simulink model "sampleModel1913_sub"  (R2023a)
settings: Solver=VariableStepAuto  StartTime=0.0  StopTime=10.0  RelTol=1e-3
libraries: hdlsllib x4, simulink x4
settings Model: Creator=user1  LastModifiedBy=user1
settings OptimizationCC: BlockReduction=off  ConditionallyExecuteInputs=off

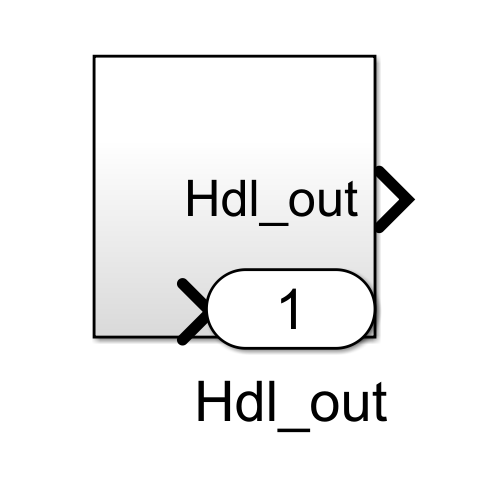
[thumbnail: Simulink's stored preview of the top-level diagram]
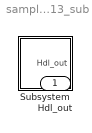
== system sampleModel1913_sub ==
  Subsystem : Subsystem
  Hdl_out : Outport  OutDataTypeStr=uint8

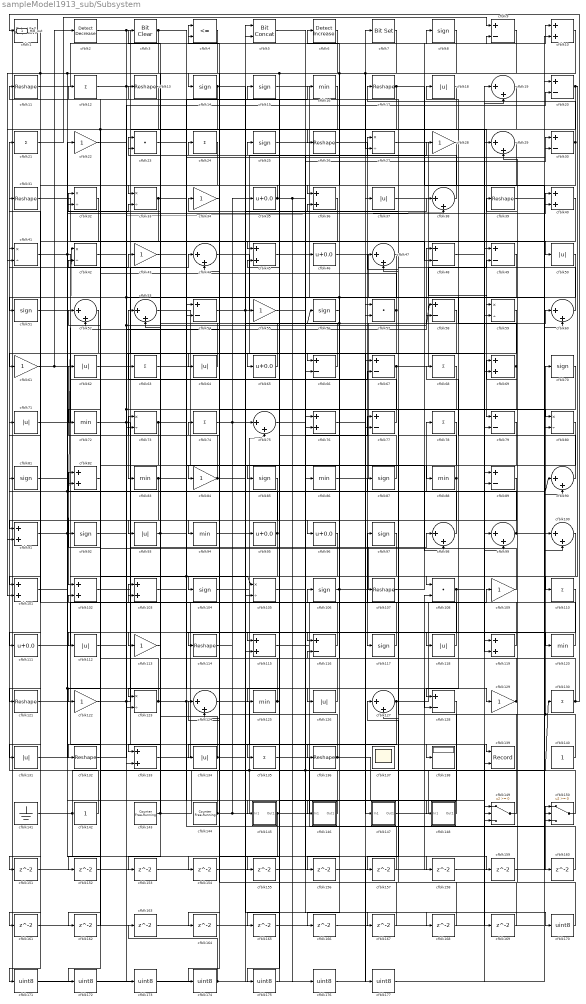
== system sampleModel1913_sub/Subsystem ==
  cfblk1 : hdlsllib/Logic and Bit Operations/Detect Fall Nonpositive  vinit=0  OutDataTypeStr=uint8
  cfblk{10,36,40,45,69,76,82,91,101..103,115,119,133} (14 alike) : Sum  OutDataTypeStr=uint8
  cfblk{19,29,38,44,47,52..53,60,75,90,98..100,124,127} (15 alike) : Sum  Inputs=|++  OutDataTypeStr=uint8
  cfblk{8,14..15,25,51,56,70,81,85,87,92,97,104,106,117} (15 alike) : Signum
  cfblk{27,32..33,41..42,59,73,80,105,123} (10 alike) : Product  Inputs=*/  OutDataTypeStr=uint8  RndMeth=Zero  SaturateOnIntegerOverflow=on
  cfblk{11,13,17,26,31,39,107,114,121,132,136} (11 alike) : Reshape
  cfblk108 : DotProduct  OutDataTypeStr=uint8
  cfblk{22,28,34,43,55,61,84,109,113,122,129} (11 alike) : Gain  OutDataTypeStr=uint8
  cfblk{12,21,24,63,68,74,78,110,130,135} (10 alike) : Sum  Inputs=+  OutDataTypeStr=uint8
  cfblk{35,46,65,95..96,111} (6 alike) : Bias  Bias=0.0  SaturateOnIntegerOverflow=off
  cfblk{18,37,50,62,64,71,93,112,118,126,131,134} (12 alike) : Abs  OutDataTypeStr=uint8  SaturateOnIntegerOverflow=off
  cfblk{9,20,30,48..49,54,58,66..67,77,79,89,116,128} (14 alike) : Sum  Inputs=+-  OutDataTypeStr=uint8
  cfblk{16,72,83,86,88,94,120,125} (8 alike) : MinMax  OutDataTypeStr=uint8
  cfblk137 : Scope
      settings: Floating=on
  cfblk138 : Display
  cfblk139 : Record  FileSettingsInternal="{\"entries\":[{\"content\":{\"excelSettings\":{\"content\":{},\"type\":\"Streamout.ExcelSettings\"}},\"type\":\"Streamout.FileSettingStorage\",\"uuid\":\"\"}],\"packageUris\":[\"http:\\/\\/schema.mathworks.com\\/mf0\\/streamout_blocks\\/R2020a\"],\"version\":\"1.0\"}"  Layout=[1 1]  SignalsInternal="{\"entries\":[{\"content\":{\"signals\":[{\"content\":{\"blockPath\":[],\"dimensions\":[1],\"domain\":\"\",\"lineColor\":\"#a2142f\",\"plots\":[1],\"port\":1,\"signalID\":51559,\"signalName\":\"cfblk72\"},\"type\":\"RecordBlkView.Signal\",\"uuid\":\"\"},{\"content\":{\"blockPath\":[],\"dimensions\":[1],\"domain\":\"\",\"lineColor\":\"#139fff\",\"plots\":[1],\"port\":2,\"signalID\":51562,\"signalName\":\"cfblk92\"},\"type\":\"RecordBlkView.Signal\",\"uuid\":\"\"}]},\"type\":\"RecordBlkView.InputSignals\",\"uuid\":\"\"}],\"packageUris\":[\"http:\\/\\/schema.mathworks.com\\/mf0\\/streamout_blocks\\/R2020a\"],\"version\":\"1.0\"}"  VisualizationBindings="{\"xyplotplugin\":{\"info\":[{\"series\":[{\"bindingParametersList\":[{\"parameter\":\"X-Axis\",\"signalID\":51559,\"signalName\":\"cfblk72\"},{\"parameter\":\"Y-Axis\",\"signalID\":51562,\"signalName\":\"cfblk92\"}],\"seriesID\":58635}],\"subplotID\":1}]}}"  CompatibilityTag=XY  st=-1
  cfblk140 : Constant  OutDataTypeStr=uint8  SampleTime=-1
  cfblk141 : Ground
  cfblk142 : Constant  OutDataTypeStr=uint8  SampleTime=-1
  cfblk143 : hdlsllib/Sources/Counter Free-Running  NumBits=16  tsamp=-1
  cfblk144 : hdlsllib/Sources/Counter Free-Running  NumBits=16  tsamp=-1
  cfblk145 : Subsystem
      settings: LibrarySourceBlock=|
      | hdlsllib/Ports &
      | Subsystems/Subsystem
  cfblk146 : Subsystem
      settings: LibrarySourceBlock=|
      | hdlsllib/Ports &
      | Subsystems/Subsystem
  cfblk147 : Subsystem
      settings: LibrarySourceBlock=|
      | hdlsllib/Ports &
      | Subsystems/Subsystem
  cfblk148 : Subsystem
      settings: LibrarySourceBlock=|
      | hdlsllib/Ports &
      | Subsystems/Subsystem
  cfblk149 : Switch  OutDataTypeStr=uint8  SaturateOnIntegerOverflow=off  InputSameDT=off
  cfblk150 : Switch  OutDataTypeStr=uint8  SaturateOnIntegerOverflow=off  InputSameDT=off
  cfblk{151..169} (19 alike) : Delay  SampleTime=1
  cfblk{170..177} (8 alike) : DataTypeConversion  OutDataTypeStr=uint8  SaturateOnIntegerOverflow=off  RndMeth=Floor
  cfblk2 : simulink/Logic and Bit Operations/Detect Decrease  vinit=0.0  OutDataTypeStr=uint8
      settings: LibrarySourceBlock=|
      | hdlsllib/Logic and Bit
      | Operations/Detect
      | Decrease
  cfblk23 : DotProduct  OutDataTypeStr=uint8
  cfblk3 : simulink/Logic and Bit Operations/Bit Clear  iBit=0
      settings: LibrarySourceBlock=|
      | hdlsllib/Logic and Bit
      | Operations/Bit Clear
  cfblk4 : RelationalOperator  Operator=<=  OutDataTypeStr=boolean  InputSameDT=off
  cfblk5 : hdlsllib/Logic and Bit Operations/Bit Concat  numInputs=2
  cfblk57 : DotProduct  OutDataTypeStr=uint8
  cfblk6 : simulink/Logic and Bit Operations/Detect Increase  vinit=0.0  OutDataTypeStr=uint8
      settings: LibrarySourceBlock=|
      | hdlsllib/Logic and Bit
      | Operations/Detect
      | Increase
  cfblk7 : simulink/Logic and Bit Operations/Bit Set  iBit=0
      settings: LibrarySourceBlock=|
      | hdlsllib/Logic and Bit
      | Operations/Bit Set
  Hdl_out : Outport  OutDataTypeStr=uint8
  wires:
  cfblk4/1 -> cfblk14/1
  cfblk72/1 -> cfblk139/1, cfblk77/2, cfblk58/2
  cfblk2/1 -> cfblk66/1, cfblk69/2, cfblk60/2
  cfblk45/1 -> cfblk86/1
  cfblk15/1 -> cfblk108/1
  cfblk114/1 -> cfblk55/1, cfblk75/1
  cfblk142/1 -> cfblk21/1
  cfblk99/1 -> cfblk90/2, cfblk6/1, cfblk56/1
  cfblk111/1 -> cfblk106/1
  cfblk64/1 -> cfblk41/1
  cfblk30/1 -> cfblk64/1, cfblk17/1
  cfblk91/1 -> cfblk159/1, cfblk42/1
  cfblk61/1 -> cfblk2/1, cfblk104/1
  cfblk26/1 -> cfblk117/1
  cfblk41/1 -> cfblk146/1(In1), cfblk138/1
  cfblk144/1 -> cfblk92/1, cfblk35/1, cfblk130/1, cfblk75/2
  cfblk149/1 -> cfblk81/1
  cfblk32/1 -> cfblk91/1
  cfblk116/1 -> cfblk71/1
  cfblk148/1(Out1) -> cfblk34/1
  cfblk122/1 -> cfblk38/2, cfblk44/1
  cfblk121/1 -> cfblk128/2, cfblk22/1
  cfblk81/1 -> cfblk102/1
  cfblk27/1 -> cfblk79/1
  cfblk86/1 -> cfblk48/1
  cfblk38/1 -> cfblk23/1
  cfblk69/1 -> cfblk165/1, cfblk18/1
  cfblk21/1 -> cfblk9/1
  cfblk85/1 -> cfblk93/1
  cfblk101/1 -> cfblk40/1
  cfblk84/1 -> cfblk60/1, cfblk62/1
  cfblk140/1 -> cfblk116/2, cfblk70/1
  cfblk34/1 -> cfblk4/1
  cfblk43/1 -> cfblk85/1
  cfblk17/1 -> cfblk73/2, cfblk40/2
  cfblk62/1 -> cfblk65/1
  cfblk97/1 -> cfblk112/1
  cfblk12/1 -> cfblk45/1, cfblk59/1
  cfblk123/1 -> cfblk42/2, cfblk145/1(In1), cfblk126/1
  cfblk105/1 -> cfblk77/1
  cfblk65/1 -> cfblk24/1
  cfblk92/1 -> cfblk139/2
  cfblk135/1 -> cfblk150/1
  cfblk133/1 -> cfblk109/1
  cfblk25/1 -> cfblk150/2
  cfblk11/1 -> cfblk8/1
  cfblk115/1 -> cfblk120/1
  cfblk6/1 -> cfblk113/1
  cfblk95/1 -> cfblk74/1, cfblk122/1
  cfblk13/1 -> cfblk41/2, cfblk132/1
  cfblk35/1 -> cfblk33/1, cfblk176/1, cfblk30/2
  cfblk57/1 -> cfblk32/2, cfblk83/1
  cfblk113/1 -> cfblk3/1
  cfblk46/1 -> cfblk100/1
  cfblk18/1 -> cfblk123/1
  cfblk141/1 -> cfblk177/1, cfblk66/2, cfblk59/2
  cfblk100/1 -> cfblk133/1
  cfblk71/1 -> cfblk37/1
  cfblk102/1 -> cfblk57/2
  cfblk14/1 -> cfblk168/1, cfblk63/1
  cfblk145/1(Out1) -> cfblk164/1, cfblk97/1
  cfblk147/1(Out1) -> cfblk19/1
  cfblk107/1 -> cfblk9/2
  cfblk67/1 -> cfblk94/1, cfblk49/2
  cfblk96/1 -> cfblk114/1
  cfblk75/1 -> cfblk28/1
  cfblk98/1 -> cfblk78/1
  cfblk10/1 -> cfblk27/2, cfblk26/1, cfblk76/2
  cfblk103/1 -> cfblk16/1
  cfblk127/1 -> cfblk134/1, cfblk19/2
  cfblk131/1 -> cfblk90/1, cfblk43/1
  cfblk77/1 -> cfblk53/1
  cfblk31/1 -> cfblk48/2
  cfblk118/1 -> cfblk23/2
  cfblk93/1 -> cfblk153/1, cfblk67/2
  cfblk82/1 -> cfblk52/1
  cfblk83/1 -> cfblk105/2, cfblk131/1
  cfblk20/1 -> cfblk124/2, cfblk110/1
  cfblk1/1 -> cfblk61/1
  cfblk150/1 -> cfblk15/1
  cfblk28/1 -> cfblk84/1
  cfblk60/1 -> cfblk11/1
  cfblk136/1 -> cfblk169/1, cfblk52/2
  cfblk120/1 -> cfblk31/1
  cfblk108/1 -> cfblk127/2, cfblk29/1
  cfblk80/1 -> cfblk135/1
  cfblk109/1 -> cfblk12/1
  cfblk23/1 -> cfblk115/1
  cfblk36/1 -> cfblk133/2
  cfblk50/1 -> cfblk121/1
  cfblk9/1 -> cfblk36/1
  cfblk63/1 -> cfblk95/1
  cfblk3/1 -> cfblk129/1, cfblk82/2, cfblk91/2
  cfblk90/1 -> cfblk68/1
  cfblk146/1(Out1) -> cfblk82/1
  cfblk19/1 -> cfblk119/2
  cfblk70/1 -> cfblk128/1
  cfblk48/1 -> cfblk50/1
  cfblk66/1 -> cfblk32/1
  cfblk51/1 -> cfblk33/2
  cfblk106/1 -> cfblk166/1, cfblk98/1
  cfblk16/1 -> cfblk72/1
  cfblk37/1 -> cfblk99/1
  cfblk134/1 -> cfblk103/1, cfblk148/1(In1)
  cfblk129/1 -> cfblk69/1, cfblk36/2
  cfblk74/1 -> cfblk136/1
  cfblk44/1 -> cfblk147/1(In1)
  cfblk124/1 -> cfblk149/2
  cfblk88/1 -> cfblk47/2, cfblk115/2
  cfblk49/1 -> cfblk88/1
  cfblk125/1 -> cfblk45/2, cfblk73/1
  cfblk87/1 -> cfblk13/1
  cfblk132/1 -> cfblk20/2, cfblk58/1
  cfblk7/1 -> cfblk174/1
  cfblk33/1 -> cfblk30/1, cfblk123/2
  cfblk143/1 -> cfblk103/2, cfblk46/1
  cfblk53/1 -> cfblk98/2
  cfblk73/1 -> cfblk172/1, cfblk118/1, cfblk105/1
  cfblk52/1 -> cfblk101/1
  cfblk29/1 -> cfblk44/2
  cfblk94/1 -> cfblk38/1
  cfblk117/1 -> cfblk107/1
  cfblk104/1 -> cfblk10/1
  cfblk79/1 -> cfblk116/1
  cfblk130/1 -> cfblk47/1, cfblk1/1
  cfblk76/1 -> cfblk80/1
  cfblk24/1 -> cfblk51/1
  cfblk47/1 -> cfblk96/1, cfblk54/2
  cfblk126/1 -> cfblk53/2
  cfblk119/1 -> cfblk87/1
  cfblk54/1 -> cfblk79/2, cfblk27/1
  cfblk8/1 -> cfblk125/1, cfblk101/2, cfblk111/1
  cfblk58/1 -> cfblk151/1
  cfblk151/1 -> cfblk76/1
  cfblk110/1 -> cfblk152/1
  cfblk152/1 -> cfblk150/3
  cfblk153/1 -> cfblk108/2
  cfblk22/1 -> cfblk154/1
  cfblk154/1 -> cfblk119/1
  cfblk128/1 -> cfblk155/1
  cfblk155/1 -> cfblk67/1
  cfblk56/1 -> cfblk156/1
  cfblk156/1 -> cfblk49/1
  cfblk68/1 -> cfblk157/1
  cfblk157/1 -> cfblk57/1
  cfblk42/1 -> cfblk158/1
  cfblk158/1 -> cfblk149/1
  cfblk159/1 -> cfblk29/2
  cfblk39/1 -> cfblk160/1
  cfblk160/1 -> cfblk54/1
  cfblk59/1 -> cfblk161/1
  cfblk161/1 -> cfblk149/3
  cfblk78/1 -> cfblk162/1
  cfblk162/1 -> cfblk102/2
  cfblk163/1 -> cfblk10/2
  cfblk164/1 -> cfblk80/2
  cfblk165/1 -> cfblk99/2
  cfblk166/1 -> cfblk20/1
  cfblk55/1 -> cfblk167/1
  cfblk167/1 -> cfblk124/1
  cfblk168/1 -> cfblk4/2
  cfblk169/1 -> cfblk127/1
  cfblk5/1 -> cfblk170/1
  cfblk170/1 -> cfblk39/1
  cfblk40/1 -> cfblk171/1
  cfblk171/1 -> cfblk5/1
  cfblk172/1 -> cfblk5/2
  cfblk112/1 -> cfblk173/1
  cfblk173/1 -> cfblk7/1
  cfblk174/1 -> Hdl_out/1, cfblk100/2, cfblk163/1
  cfblk89/1 -> cfblk175/1
  cfblk175/1 -> cfblk25/1
  cfblk176/1 -> cfblk89/1
  cfblk177/1 -> cfblk89/2

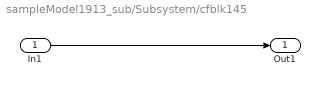
== system sampleModel1913_sub/Subsystem/cfblk145 ==
  In1 : Inport
  Out1 : Outport
  wires:
  In1/1 -> Out1/1

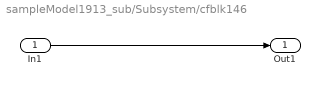
== system sampleModel1913_sub/Subsystem/cfblk146 ==
  In1 : Inport
  Out1 : Outport
  wires:
  In1/1 -> Out1/1

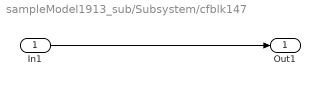
== system sampleModel1913_sub/Subsystem/cfblk147 ==
  In1 : Inport
  Out1 : Outport
  wires:
  In1/1 -> Out1/1

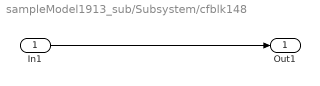
== system sampleModel1913_sub/Subsystem/cfblk148 ==
  In1 : Inport
  Out1 : Outport
  wires:
  In1/1 -> Out1/1
